simulink model "lift"  (R2020a)
settings: Solver=VariableStepAuto  StartTime=0.0  StopTime=10.0  RelTol=1e-3
settings Model: Creator=kasutav  LastModifiedBy=kasutav

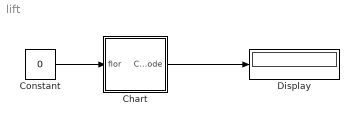
== system lift ==
  Chart : Stateflow chart  TreatAsAtomicUnit=on
  Constant : Constant  Value=0
  Display : Display
  wires:
  Constant/1 -> Chart/1(flor)
  Chart/1(ChartMode) -> Display/1

== stateflow chart lift/Chart ==
  state First
    en:
    %flor=1
    du:
    after(3)
    flor=2
  state Second
    en:
    flor=2
    du:
    after(3)
    flor=3
  state Ground
    en:
    %flor=0
    du:
    after(3)
    flor=1
  state Third
    en:
    after(3)
    flor=4
  state Fourth
    en:
    after(3)
    flor=3
  (default) -> Ground
  First -> Second : [flor==2]
  Ground -> First : [flor==1]
  Second -> Third : [flor==3]
  Third -> Fourth : [flor==4]
  Fourth -> Third : [flor==3]
  data: ChartMode output Enum: ChartModeType; flor input
